simulink model "Progetto_b3_simulink_gruppoM"  (R2021a)
settings: Solver=VariableStepAuto  StartTime=0.0  StopTime=10.0  RelTol=1e-3
InitFcn:
  | beta1 = 0.25; % [N/m^2] Coefficiente di attrito
  | beta2 = 2.5; % [N/m^2] Coefficiente di attrito
  | m = 250; % [kg] Massa
  | k = 3.5; % Parametro adimensionale
  | rho_e = 3e8; % [m] Distanza tra terra e satellite
  | k_g = 6.67e-11; % [N*m^2/kg] Costante di gravitazione universale
  | M = 5.98e24; % [kg] Massa della Terra
  | %Matrici all'equilibrio
  | A_e = [0,                                                          1,                      0;
  |      (k-1)*((-3*k_g*M)/(rho_e^3)),                           -beta1/m,        -2*(k-1)*sqrt((k_g*M)/rho_e);
  |      -(beta2/(m*(rho_e^2)))*sqrt((k_g*M)/rho_e), -(2/rho_e)*sqrt((k_g*M)/(rho_e^3)), -beta2/m];
  | 
  | B_e = [0; 0; 1/(m*rho_e)];
  | 
  | C_e = [0, 0, 1];
  | 
  | D_e = 0;
  | 
  | u_e = beta2*sqrt((k_g*M)/rho_e);
  | x3_e = sqrt((k_g*M)/(rho_e^3));
values from neighbouring files (symbols this model uses):
  omega_d = 0.125    [Progetto_b3_Matlab_gruppoM.m]
  omega_n = 2.5e4    (= 25000)    [Progetto_b3_Matlab_gruppoM.m]
  RR_d = mu_d*RR_a    [Progetto_b3_Matlab_gruppoM.m]
  RR_s = mu_s / s    [Progetto_b3_Matlab_gruppoM.m]
  x_e = [x1_e; x2_e; x3_e]    [Progetto_b3_Matlab_gruppoM.m]
libraries: cstblocks x1
settings Model: Creator=ubolakes  LastModifiedBy=ubolakes

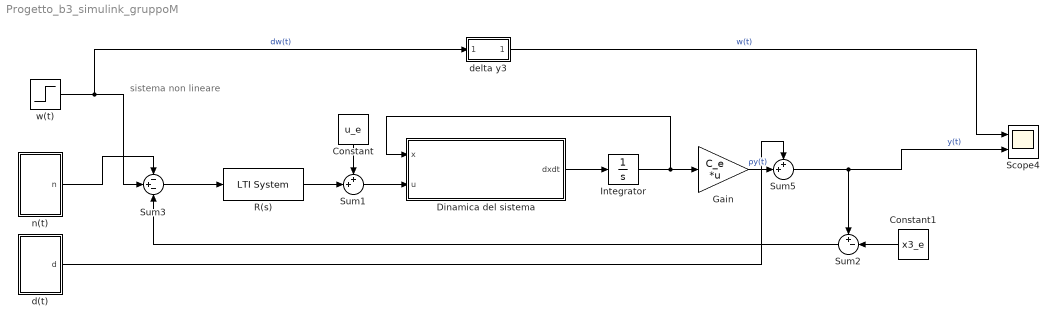
== system Progetto_b3_simulink_gruppoM ==
  note: sistema non lineare
  Constant : Constant  Value=u_e
  Constant1 : Constant  Value=x3_e
  Dinamica del sistema : MATLAB Function  TreatAsAtomicUnit=on
  Gain : Gain  Gain=C_e  Multiplication=Matrix(K*u)
  Integrator : Integrator  InitialCondition=x_e
  R(s) : cstblocks/LTI System  sys=RR_s*RR_d  IC=[]
  Scope4 : Scope  NumInputPorts=2
  Sum1 : Sum  Inputs=++|
  Sum2 : Sum  Inputs=+-|
  Sum3 : Sum  Inputs=-+-
  Sum5 : Sum  Inputs=++|
  d(t) : Subsystem
  delta y3 : Subsystem
  n(t) : Subsystem
  w(t) : Step  Time=2  After=-3e-7  SampleTime=0
  wires:
  w(t)/1 -> Sum3/2, delta y3/1(In1)  "dw(t)"
  delta y3/1(Out1) -> Scope4/1  "w(t)"
  Sum5/1 -> Scope4/2, Sum2/1  "y(t)"
  d(t)/1(d) -> Sum5/1
  Gain/1 -> Sum5/2  "ρy(t)"
  n(t)/1(n) -> Sum3/1
  Constant/1 -> Sum1/1
  Dinamica del sistema/1(dxdt) -> Integrator/1
  Sum1/1 -> Dinamica del sistema/2(u)
  Sum3/1 -> R(s)/1
  R(s)/1 -> Sum1/2
  Sum2/1 -> Sum3/3
  Constant1/1 -> Sum2/2
  Integrator/1 -> Dinamica del sistema/1(x), Gain/1

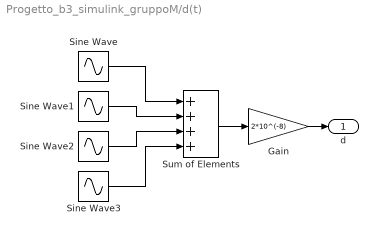
== system Progetto_b3_simulink_gruppoM/d(t) ==
  Gain : Gain  Gain=2*10^(-8)
  Sine Wave : Sin  Frequency=omega_d  SampleTime=0
  Sine Wave1 : Sin  Frequency=2*omega_d  SampleTime=0
  Sine Wave2 : Sin  Frequency=3*omega_d  SampleTime=0
  Sine Wave3 : Sin  Frequency=4*omega_d  SampleTime=0
  Sum of Elements : Sum  Inputs=++++  InputSameDT=on
  d : Outport
  wires:
  Sum of Elements/1 -> Gain/1
  Sine Wave2/1 -> Sum of Elements/3
  Gain/1 -> d/1
  Sine Wave/1 -> Sum of Elements/1
  Sine Wave3/1 -> Sum of Elements/4
  Sine Wave1/1 -> Sum of Elements/2

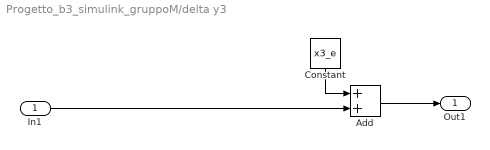
== system Progetto_b3_simulink_gruppoM/delta y3 ==
  In1 : Inport
  Add : Sum
  Constant : Constant  Value=x3_e
  Out1 : Outport
  wires:
  In1/1 -> Add/2
  Constant/1 -> Add/1
  Add/1 -> Out1/1

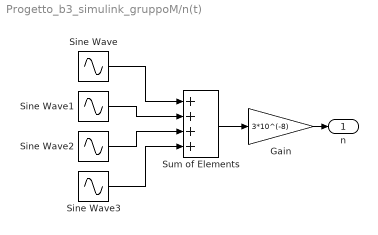
== system Progetto_b3_simulink_gruppoM/n(t) ==
  Gain : Gain  Gain=3*10^(-8)
  Sine Wave : Sin  Frequency=omega_n  SampleTime=0
  Sine Wave1 : Sin  Frequency=2*omega_n  SampleTime=0
  Sine Wave2 : Sin  Frequency=3*omega_n  SampleTime=0
  Sine Wave3 : Sin  Frequency=4*omega_n  SampleTime=0
  Sum of Elements : Sum  Inputs=++++  InputSameDT=on
  n : Outport
  wires:
  Sum of Elements/1 -> Gain/1
  Sine Wave2/1 -> Sum of Elements/3
  Gain/1 -> n/1
  Sine Wave/1 -> Sum of Elements/1
  Sine Wave3/1 -> Sum of Elements/4
  Sine Wave1/1 -> Sum of Elements/2

== matlab function Progetto_b3_simulink_gruppoM/Dinamica del sistema ==
  data: x input; u input; dxdt output
function dxdt = systemDynamics(x,u)
beta1 = 0.25; % [N/m^2] Coefficiente di attrito
beta2 = 2.5; % [N/m^2] Coefficiente di attrito
m = 250; % [kg] Massa
k = 3.5; % Parametro adimensionale
k_g = 6.67e-11; % [N*m^2/kg] Costante di gravitazione universale
M = 5.98e24; % [kg] Massa della Terra

dx1dt=x(2);
dx2dt=-beta1*x(2)/m+(k-1)*(k_g*M/(x(1)^2) - x(1)*(x(3)^2));
dx3dt=-2*x(3)*x(2)/x(1)-beta2*x(3)/m+u/(m*x(1));

dxdt = [dx1dt; dx2dt; dx3dt;];
